simulink model "hardware_IOTest"  (R2022b)
settings: Solver=FixedStepAuto  StartTime=0.0  StopTime=inf  FixedStep=1/30  RelTol=1e-3  EnableMultiTasking=on
undefined symbols (not defined in the file): qc_get_step_size
libraries: quarc_library x4
settings Model: SimulationMode=external  Creator=kfullerton  LastModifiedBy=Kelly Fullerton
settings SolverCC: PositivePriorityOrder=on
settings HardwareCC: ProdBitPerLong=64  ProdLargestAtomicInteger=LongLong  ProdLargestAtomicFloat=Double  ProdLongLongMode=on  ProdHWDeviceType=ARM Compatible->ARM 64-bit (LP64)
settings ModelReferenceCC: EnableRefExpFcnMdlSchedulingChecks=on
settings RTWCC: Description=QUARC Linux Raspberry Pi Arm64 Target (QBot Platform) Using Toolchain  SystemTargetFile=quarc_linux_pi_arm64.tlc  Toolchain=QUARC linux_pi_arm64 | gmake (64-bit Windows)  BuildConfiguration=Faster Runs
settings STFCustomTargetCC: TargetLangStandard=C99 (ISO)  ConcurrentExecutionCompliant=on  GRTInterface=on  UseToolchainInfoCompliant=on  SystemTargetFile=quarc_linux_pi_arm64.tlc
settings GRTTargetCC: ParMdlRefBuildCompliant=off  CompOptLevelCompliant=off  CombineOutputUpdateFcns=off  MatFileLogging=off  CPPClassGenCompliant=off  GRTInterface=on  ExtMode=on  ExtModeMexFile=quarc_comm  ExtModeMexArgs='-w -d /tmp -uri %u','tcpip://192.168.2.X:17002'

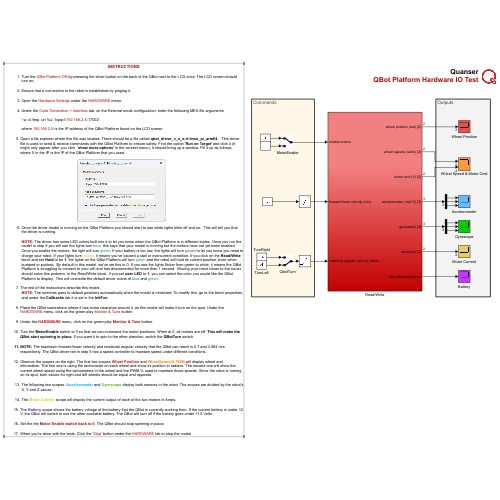
[thumbnail: Simulink's stored preview of the top-level diagram]
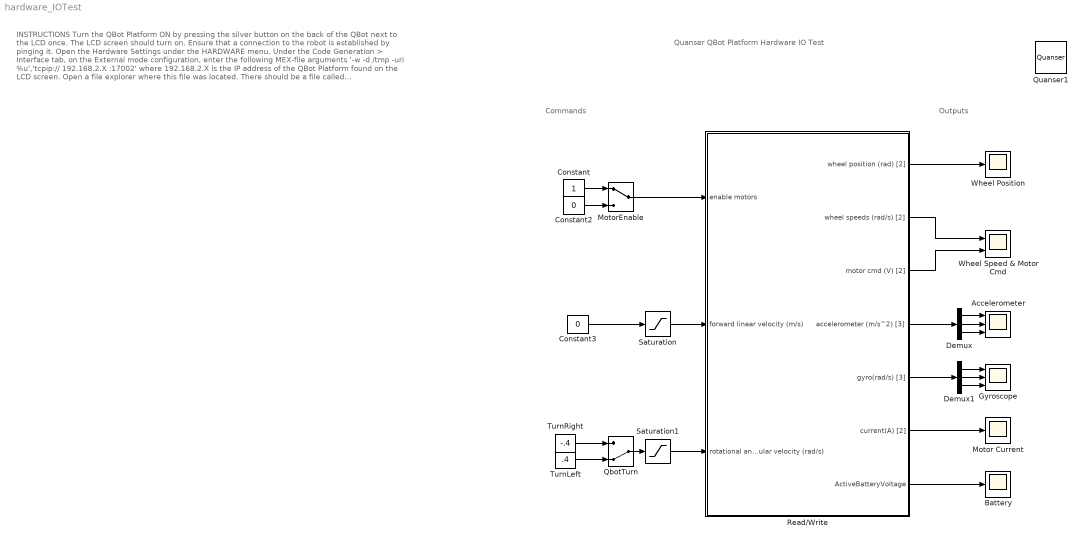
== system hardware_IOTest ==
  note: Outputs
  note: Commands
  note: INSTRUCTIONS
      |
      | Turn the QBot Platform ON by pressing the silver button on the back of the QBot next to the LCD once. The LCD screen should turn on.
      |
      | Ensure that a connection to the robot is established by pinging it.
      |
      | Open the Hardware Settings under the HARDWARE menu.
      |
      | Under the Code Generation > Interface tab, on the External mode configuration, enter the following MEX-file arguments
      |
      | '-w -d /tmp -uri %u','tcpip:// 192.168.2.X :17002'
      |
      | where 192.168.2.X is the IP address of the QBot Platform found on the LCD screen.
      |
      | Open a file explorer where this file was located. There should be a file called qbot_driver_v_x_x.rt-linus_pi_arm64 . This driver file is used to send & receive commands with the QBot Platform to ensure safety. Find the option ' Run on Target ' and click it (it might only appear after you click ' show more options ' in the context menu). It should bring up a window. Fill it up as follows; where X in the IP is the IP of the QBot Platform that you used.
      |
      | Once the driver model is running on the QBot Platform you should start to see white lights blink off and on. This will tell you that the driver is running.
      |
      | NOTE: The driver has some LED colors built into it to let you know when the QBot Platform is in different states. Once you run the model in step 9 you will see the lights turn blue , this says that your model is running but the motors have not yet been enabled. Once you enable the motors, the light will turn green . If your battery is too low, the lights will turn purple to let you know you need to charge your robot. If your lights turn yellow , it means you've caused a stall or overcurrent condition. If you click on the Read/Write block and set Hold to be 1 , the lights on the QBot Platform will turn green and the robot will hold its current position, even when bumped or pushed. By default in this model, we've set this to 0. If you see the lights flicker from green to white, it means the QBot Platform is struggling to connect to your wifi and has disconnected for more then 1 second. Moving your robot closer to the router should solve this problem. In the Read/Write block, if you set user LED to 1 , you can select the color you would like the QBot Platform to display. This will overwrite the default driver colors of blue and green .
      |
      | The rest of the instructions describe this model.
      | NOTE: The switches goes to default positions automatically when the model is initialized. To modify this, go to the block properties, and under the Callbacks tab it is set in the InitFcn .
      |
      | Place the QBot somewhere where it has some clearance around it, as this model will make it turn on the spot. Under the HARDWARE menu, click on the green play Monitor & Tune button.
      |
      | Under the HARDWARE menu, click on the green play Monitor & Tune button.
      |
      | Turn the MotorEnable switch to 1 so that we can command the motor positions. When at 0, all motors are off. This will make the QBot start spinning in place. If you want it to spin to the other direction, switch the QBotTurn switch.
      |
      | NOTE: The maximum forward linear velocity and rotational angular velocity that the QBot can reach is 0.7 and 3.564 m/s respectively. The QBot driver ran in step 5 has a speed controller to maintain speed under different conditions.
      |
      | Observe the scopes on the right. The first two scopes Wheel Position and WheelSpeed & PWM will display wheel and information. The first one is using the tachometer on each wheel and show its position in radians. The second one will show the current wheel speed using the tachometers in the wheel and the PWM % used to maintain those speeds. Since the robot is turning on its spot, both values for right and left wheels should be equal and opposite.
      |
      | The following two scopes, Accelerometer and Gyroscope display both sensors in the robot. The scopes are divided by the robot's X, Y and Z values.
      |
      | The Motor Current scope will display the current output of each of the two motors in Amps.
      |
      | The Battery scope shows the battery voltage of the battery that the QBot is currently working from. If the current battery is under 12 V, the QBot will switch to use the other available battery. The QBot will turn off if the battery goes under 11.5 Volts.
      |
      | Set the the Motor Enable switch back to 0 . The QBot should stop spinning in place.
      |
      | When you're done with the tests, Click the ' Stop ' button under the HARDWARE tab to stop the model.
  note: Quanser
      | QBot Platform Hardware IO Test
  Accelerometer : Scope  NumInputPorts=3
  Battery : Scope
  Constant : Constant
  Constant2 : Constant  Value=0
  Constant3 : Constant  Value=0
  Demux : Demux  Outputs=3
  Demux1 : Demux  Outputs=3
  Gyroscope : Scope  NumInputPorts=3
  Motor Current : Scope
  MotorEnable : ManualSwitch  InitFcn=set_param(gcb,'sw','0')
  QbotTurn : ManualSwitch  CurrentSetting=0
  Quanser1 : quarc_library/Logos/Quanser
  Read/Write : Subsystem
  Saturation : Saturate  UpperLimit=0.7  LowerLimit=-0.7
  Saturation1 : Saturate  UpperLimit=3.564  LowerLimit=-3.564
  TurnLeft : Constant  Value=.4
  TurnRight : Constant  Value=-.4
  Wheel Position : Scope
  Wheel Speed & Motor Cmd : Scope  NumInputPorts=2
  wires:
  MotorEnable/1 -> Read/Write/1(enable motors)
  Constant/1 -> MotorEnable/1
  Constant3/1 -> Saturation/1
  QbotTurn/1 -> Saturation1/1
  TurnRight/1 -> QbotTurn/1
  TurnLeft/1 -> QbotTurn/2
  Read/Write/2(wheel speeds (rad/s) [2]) -> Wheel Speed & Motor Cmd/1
  Read/Write/3(motor cmd (V) [2]) -> Wheel Speed & Motor Cmd/2
  Read/Write/1(wheel position (rad) [2]) -> Wheel Position/1
  Read/Write/4(accelerometer (m/s^2) [3]) -> Demux/1
  Demux/1 -> Accelerometer/1
  Demux/2 -> Accelerometer/2
  Demux/3 -> Accelerometer/3
  Demux1/1 -> Gyroscope/1
  Read/Write/5(gyro(rad/s) [3]) -> Demux1/1
  Demux1/3 -> Gyroscope/3
  Demux1/2 -> Gyroscope/2
  Read/Write/6(current(A) [2]) -> Motor Current/1
  Read/Write/7(ActiveBatteryVoltage) -> Battery/1
  Constant2/1 -> MotorEnable/2
  Saturation/1 -> Read/Write/2(forward linear velocity (m/s))
  Saturation1/1 -> Read/Write/3(rotational angular velocity (rad/s))

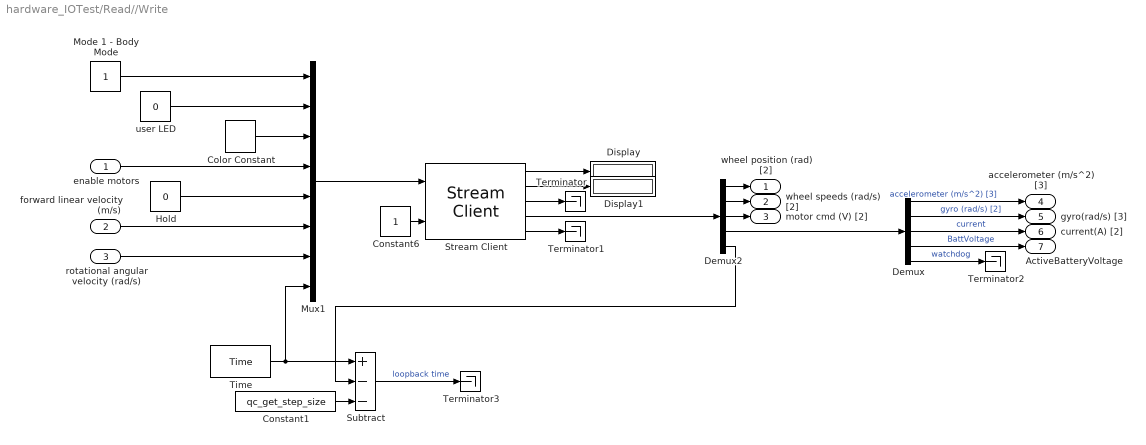
== system hardware_IOTest/Read//Write ==
  enable motors : Inport
  forward linear velocity (m/s) : Inport  Port=2
  rotational angular velocity (rad/s) : Inport  Port=3
  Color Constant : quarc_library/Sources/Signals/Color Constant  color=[0 1 1]
      settings: SourceProductName=QUARC Targets
  Constant1 : Constant  Value=qc_get_step_size
  Constant6 : Constant
  Demux : Demux  Outputs=[3 3 2 1 1]
  Demux2 : Demux  Outputs=[2 2 2 10 1]
  Display : Display
  Display1 : Display
  Hold : Constant  Value=0
  Mode 1 - Body Mode : Constant
  Mux1 : Mux  Inputs=8
  Stream Client : quarc_library/Communications/Basic/Stream Client  uri_source=Specify via dialog (do not evaluate)  uri=tcpip://localhost:18888  send_buffer_size=1460  receive_buffer_size=1460  byte_order=little endian (Intel - LSB first)  optimization=Minimum latency  send_options=Send most recent data  receive_options=Receive most recent data  default_value=zeros(17,1)  sample_time=qc_get_step_size  active=off  implementation=Use blocking I/O in a separate thread  send_fifo_size=1000  receive_fifo_size=1000  send_priority=0  receive_priority=0  send_dimensions=off  receive_dimensions=off  max_dimensions=-1  data_type=Inherited via back propagation  type_expr=BusObject
      settings: AttributesFormatString="\"tcpip://localhost:18888\""
  Subtract : Sum  Inputs=+--
  Terminator{,1..3} (4 alike) : Terminator
  Time : quarc_library/Sources/Time/Time  time_source=Wall clock  sample_time=qc_get_step_size
  user LED : Constant  Value=0
  wheel position (rad) [2] : Outport
  wheel speeds (rad/s) [2] : Outport  Port=2
  motor cmd (V) [2] : Outport  Port=3
  accelerometer (m/s^2) [3] : Outport  Port=4
  gyro(rad/s) [3] : Outport  Port=5
  current(A) [2] : Outport  Port=6
  ActiveBatteryVoltage : Outport  Port=7
  wires:
  Stream Client/5 -> Terminator1/1
  Mode 1 - Body Mode/1 -> Mux1/1
  user LED/1 -> Mux1/2
  enable motors/1 -> Mux1/4
  Demux2/4 -> Demux/1
  Mux1/1 -> Stream Client/1
  Stream Client/2 -> Display1/1
  Stream Client/4 -> Demux2/1
  Stream Client/1 -> Display/1
  forward linear velocity (m/s)/1 -> Mux1/6
  Color Constant/1 -> Mux1/3
  Time/1 -> Mux1/8, Subtract/1
  Constant6/1 -> Stream Client/2
  Subtract/1 -> Terminator3/1  "loopback time"
  Stream Client/3 -> Terminator/1
  Constant1/1 -> Subtract/3
  Demux2/5 -> Subtract/2
  Demux2/3 -> motor cmd (V) [2]/1
  Demux2/1 -> wheel position (rad) [2]/1
  Demux2/2 -> wheel speeds (rad/s) [2]/1
  rotational angular velocity (rad/s)/1 -> Mux1/7
  Demux/1 -> accelerometer (m/s^2) [3]/1  "accelerometer (m/s^2) [3]"
  Demux/2 -> gyro(rad/s) [3]/1  "gyro (rad/s) [2]"
  Demux/4 -> ActiveBatteryVoltage/1  "BattVoltage"
  Demux/3 -> current(A) [2]/1  "current"
  Hold/1 -> Mux1/5
  Demux/5 -> Terminator2/1  "watchdog"
